simulink model "longModel_V0_1"  (R2023a)
settings: Solver=VariableStepAuto  StartTime=0.0  StopTime=100  RelTol=1e-3  AbsTol=1e-3
undefined symbols (not defined in the file or in its folder): STire
libraries: fl_lib x14, nesl_utility x10, sdl_lib x4, simulink x1
settings Model: Creator=Raheel Farouk  LastModifiedBy=Raheel Farouk
settings SolverCC: AutoScaleAbsTol=off  AlgebraicLoopSolver=TrustRegion  MaxZcPerStep=1
settings DebuggingCC: UnconnectedInputMsg=warning  UnconnectedOutputMsg=warning  UnconnectedLineMsg=warning  SymbolicDimsDataTypeCodeGenerationDiagnostic=none
settings ModelReferenceCC: EnableRefExpFcnMdlSchedulingChecks=on
settings SFSimCC: CustomCodeUndefinedFunction=UseInterfaceOnly
settings RTWCC: DLArmComputeVersion=19.05
settings SimscapeCC: SimscapeLogType=all  SimscapeLogSimulationStatistics=on  SimscapeLogDataHistory=10000

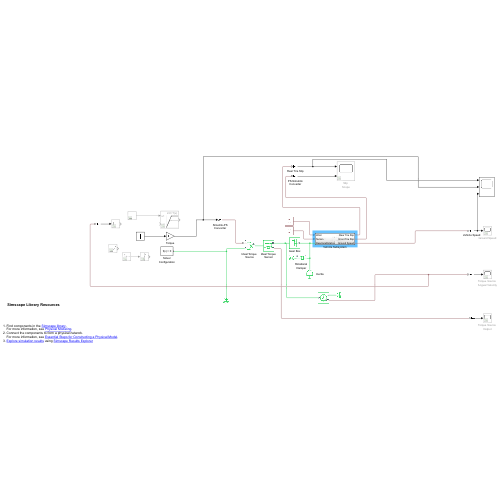
[thumbnail: Simulink's stored preview of the top-level diagram]
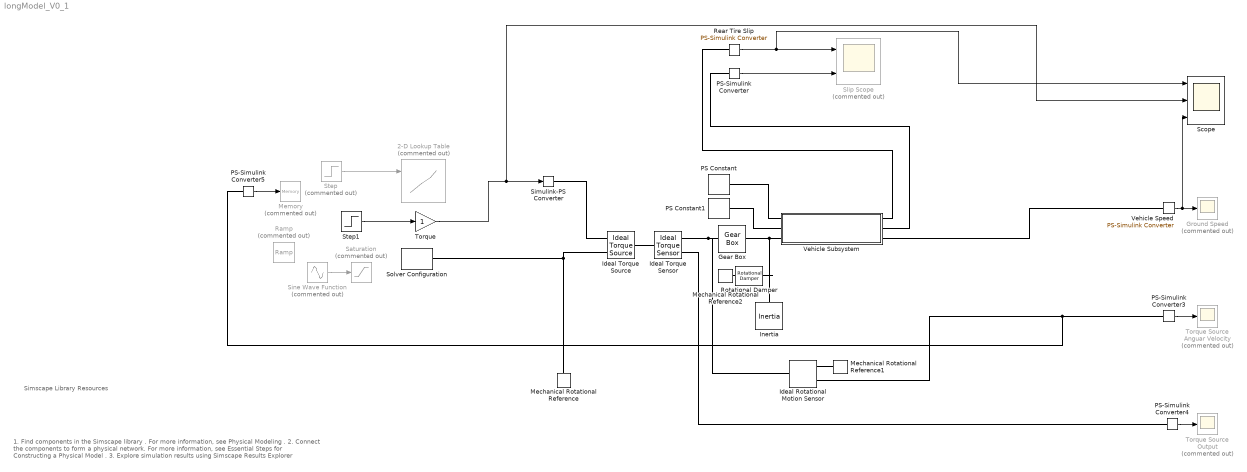
== system longModel_V0_1 ==
  note: 1. Find components in the Simscape library .
      | For more information, see Physical Modeling .
      | 2. Connect the components to form a physical network.
      | For more information, see Essential Steps for Constructing a Physical Model .
      | 3. Explore simulation results using Simscape Results Explorer
  note: Simscape Library Resources
  2-D Lookup Table : Lookup_n-D  Commented=on  BreakpointsForDimension1=[0;141;216.67;220;230;500]  BreakpointsForDimension2=[1;100;3321;5100]  Table=[0 0 0 0;141 141 141 141;216.67 216.67 216.67 141;220 220 216.67 141;220 230 216.67 141;220 230 216.67 141]  InternalRulePriority=Speed  RndMeth=Simplest
      settings: InputPortMap=u0,u1
  Gear Box : fl_lib/Mechanical/Mechanisms/Gear Box  ratio=3.15  t_in_specify=off  t_in_priority=None  t_in=0 N*m  t_in_nominal_specify=off  t_in_nominal_unit=N*m  t_in_nominal_value=1  t_out_specify=off  t_out_priority=None  t_out=0 N*m  t_out_nominal_specify=off  t_out_nominal_unit=N*m  t_out_nominal_value=1
  Ground Speed : Scope  Commented=on
  Ideal Rotational Motion Sensor : fl_lib/Mechanical/Mechanical Sensors/Ideal Rotational Motion Sensor  reference=foundation.enum.MeasurementReference.difference  acceleration_port=false  velocity_port=true  position_port=false  wrap_angle=false  offset=0 rad
      settings: InternalSimscapePortConfiguration="{\"Bottom\":[],\"Left\":[{\"id\":\"R\",\"label\":\"R\",\"type\":\"foundation.mechanical.rotational.rotational\"}],\"Right\":[{\"id\":\"C\",\"label\":\"C\",\"type\":\"foundation.mechanical.rotational.rotational\"},{\"id\":\"W\",\"label\":\"W\",\"type\":\"output\"}],\"Top\":[]}"
  Ideal Torque Sensor : fl_lib/Mechanical/Mechanical Sensors/Ideal Torque Sensor
  Ideal Torque Source : fl_lib/Mechanical/Mechanical Sources/Ideal Torque Source
  Inertia : fl_lib/Mechanical/Rotational Elements/Inertia  inertia=0.01 kg*m^2  num_ports=foundation.enum.numPorts2.one  w_specify=off  w_priority=High  w=0 rad/s  w_nominal_specify=off  w_nominal_unit=rad/s  w_nominal_value=1  t_specify=off  t_priority=None  t=0 N*m  t_nominal_specify=off  t_nominal_unit=N*m  t_nominal_value=1
  Mechanical Rotational Reference : fl_lib/Mechanical/Rotational Elements/Mechanical Rotational Reference
  Mechanical Rotational Reference1 : fl_lib/Mechanical/Rotational Elements/Mechanical Rotational Reference
  Mechanical Rotational Reference2 : fl_lib/Mechanical/Rotational Elements/Mechanical Rotational Reference
  Memory : Memory  Commented=on
  PS Constant : fl_lib/Physical Signals/Sources/PS Constant  constant=0
  PS Constant1 : fl_lib/Physical Signals/Sources/PS Constant  constant=0
  PS-Simulink Converter : nesl_utility/PS-Simulink Converter  PhysicalDomain=network_engine_domain  SubClassName=ps_output  LeftPortType=input  RightPortType=output  PseudoPeriodic=off  Frequencies=[]  VectorFormat=inherit  Unit=inherit  AffineConversion=off
  PS-Simulink Converter3 : nesl_utility/PS-Simulink Converter  PhysicalDomain=network_engine_domain  SubClassName=ps_output  LeftPortType=input  RightPortType=output  PseudoPeriodic=off  Frequencies=[]  VectorFormat=inherit  Unit=rpm  AffineConversion=off
  PS-Simulink Converter4 : nesl_utility/PS-Simulink Converter  PhysicalDomain=network_engine_domain  SubClassName=ps_output  LeftPortType=input  RightPortType=output  PseudoPeriodic=off  Frequencies=[]  VectorFormat=inherit  Unit=inherit  AffineConversion=off
  PS-Simulink Converter5 : nesl_utility/PS-Simulink Converter  PhysicalDomain=network_engine_domain  SubClassName=ps_output  LeftPortType=input  RightPortType=output  PseudoPeriodic=off  Frequencies=[]  VectorFormat=inherit  Unit=rpm  AffineConversion=off
  Ramp : simulink/Sources/Ramp  Commented=on  slope=10  start=5  InitialOutput=0
  Rear Tire Slip : nesl_utility/PS-Simulink Converter  PhysicalDomain=network_engine_domain  SubClassName=ps_output  LeftPortType=input  RightPortType=output  PseudoPeriodic=off  Frequencies=[]  VectorFormat=inherit  Unit=inherit  AffineConversion=off
  Rotational Damper : fl_lib/Mechanical/Rotational Elements/Rotational Damper  D=0.001 N*m*s/rad  w_specify=off  w_priority=None  w=0 rad/s  w_nominal_specify=off  w_nominal_unit=rad/s  w_nominal_value=1  t_specify=off  t_priority=None  t=0 N*m  t_nominal_specify=off  t_nominal_unit=N*m  t_nominal_value=1
  Saturation : Saturate  Commented=on  UpperLimit=300  LowerLimit=0
  Scope : Scope  NumInputPorts=3
  Simulink-PS Converter : nesl_utility/Simulink-PS Converter  PhysicalDomain=network_engine_domain  SubClassName=ps_input  LeftPortType=input  RightPortType=output  PseudoPeriodic=off  Frequencies=[]  NoiseDistribution=none  NoiseParameters=[]  Unit=1  AffineConversion=off  FilteringAndDerivatives=filter  SimscapeFilterOrder=1  InputFilterTimeConstant=0.001  UdotUserProvided=0
  Sine Wave Function : Sin  Commented=on  Bias=112  Frequency=0.4  SampleTime=0
  Slip Scope : Scope  Commented=on  NumInputPorts=2
  Solver Configuration : nesl_utility/Solver Configuration  PhysicalDomain=network_engine_domain  SubClassName=solver  LeftPortType=input  RightPortType=generic  Tones=[]  Harmonics=[]  SimulateNoise=off  Profile=off  UseLocalSampling=off  EnableSwitchedLinearOptims=on  FrequencyDomain=off  UseCCode=off  RelTol=0.001  AbsTol=1e-06  MinStep=1e-09  ToWorkspace=off  RevertToSquareIcSolve=off  NumHomotopyIterations=100  PhasorMode=off  PhasorModeNumHarmonics=1  ConsistencySolver=NEWTON_XTOL_AFTER_FTOL  IndexReductionMethod=DerivativeReplacement  DoDC=off  ResidualTolerance=1e-09  ConsistencyTolSource=GLOBAL  ConsistencyAbsTol=0.001  ConsistencyRelTol=0.001  ConsistencyTolFactor=0.001  UseLocalSolver=off  LocalSolverChoice=NE_BACKWARD_EULER_ADVANCER  ResolveIndetEquations=on  FunctionEvalNumThread=1  LocalSolverSampleTime=0.001  DoFixedCost=off  MaxNonlinIter=3  MaxModeIter=2  ComputeImpulses=off  ImpulseIterations=2  LinearAlgebra=auto  LinearAlgebraNumThread=0  EquationFormulation=NE_TIME_EF  DelaysMemoryBudget=1024  AutomaticFiltering=on  FilteringTimeConstant=0.001  PartitionStorageMethod=AS_NEEDED  PartitionMemoryBudget=1024  PartitionMethod=ROBUST
  Step : Step  Commented=on  Time=5  After=500  SampleTime=0
  Step1 : Step  Time=5  After=10  SampleTime=0
  Torque : Gain
  Torque Source Anguar Velocity : Scope  Commented=on
  Torque Source Output : Scope  Commented=on
  Vehicle Speed : nesl_utility/PS-Simulink Converter  PhysicalDomain=network_engine_domain  SubClassName=ps_output  LeftPortType=input  RightPortType=output  PseudoPeriodic=off  Frequencies=[]  VectorFormat=inherit  Unit=km/hr  AffineConversion=off
  Vehicle Subsystem : Subsystem
  wires:
  PS-Simulink Converter/1 -> Slip Scope/2
  Rear Tire Slip/1 -> Scope/1, Slip Scope/1
  Vehicle Speed/1 -> Scope/3, Ground Speed/1
  PS-Simulink Converter4/1 -> Torque Source Output/1
  PS-Simulink Converter3/1 -> Torque Source Anguar Velocity/1
  PS-Simulink Converter5/1 -> Memory/1
  Step/1 -> 2-D Lookup Table/1
  Sine Wave Function/1 -> Saturation/1
  Torque/1 -> Scope/2, Simulink-PS Converter/1
  Step1/1 -> Torque/1
  connections:
  Rear Tire Slip/LConn1 -- Vehicle Subsystem/RConn1
  Vehicle Subsystem/RConn2 -- PS-Simulink Converter/LConn1
  Vehicle Subsystem/RConn3 -- Vehicle Speed/LConn1
  Ideal Torque Source/RConn2 -- Solver Configuration/RConn1 -- Mechanical Rotational Reference/LConn1
  Ideal Torque Sensor/LConn1 -- Ideal Torque Source/LConn1
  PS-Simulink Converter4/LConn1 -- Ideal Torque Sensor/RConn2
  Ideal Rotational Motion Sensor/RConn1 -- Mechanical Rotational Reference1/LConn1
  Ideal Rotational Motion Sensor/RConn2 -- PS-Simulink Converter5/LConn1 -- PS-Simulink Converter3/LConn1
  PS Constant/RConn1 -- Vehicle Subsystem/LConn1
  PS Constant1/RConn1 -- Vehicle Subsystem/LConn2
  Ideal Rotational Motion Sensor/LConn1 -- Ideal Torque Sensor/RConn1 -- Gear Box/LConn1
  Vehicle Subsystem/LConn3 -- Rotational Damper/RConn1 -- Inertia/LConn1 -- Gear Box/RConn1
  Mechanical Rotational Reference2/LConn1 -- Rotational Damper/LConn1
  Simulink-PS Converter/RConn1 -- Ideal Torque Source/RConn1

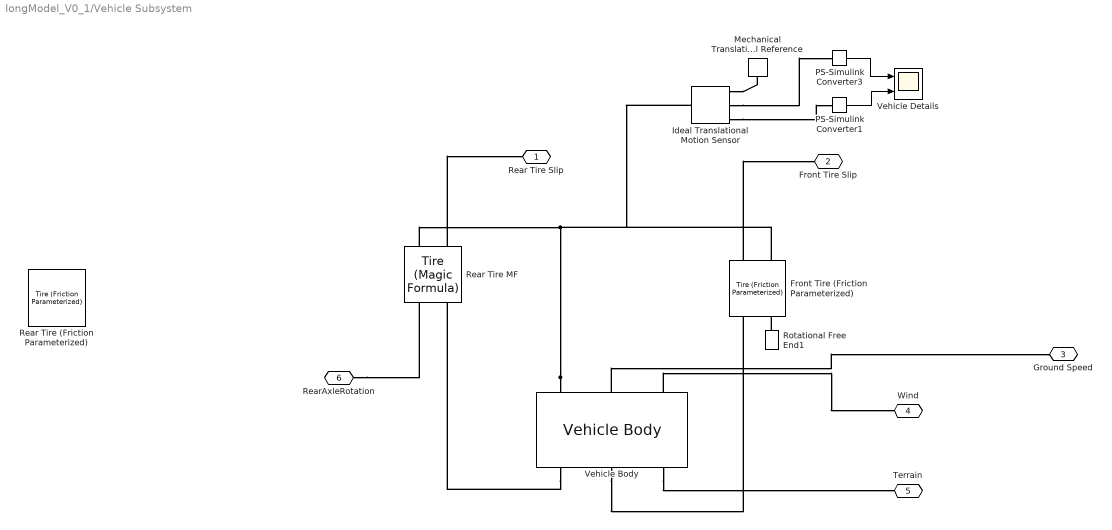
== system longModel_V0_1/Vehicle Subsystem ==
  Front Tire (Friction Parameterized) : sdl_lib/Tires & Vehicles/Tire (Friction Parameterized)  r_tire=508 mm  slip_output=sdl.enum.SlipOutput.Relative  friction_model=sdl.enum.friction_model_var.fixed  mu_static=0.9  mu_kinetic=0.7  slip_vector=[0, .02, .06, .15, .6, 1] rad/s  mu_kinetic_vector=[.89, .88, .8, .75, .7, .7]  interp_method=simscape.enum.interpolation.linear  extrap_method=simscape.enum.extrapolation.linear  model_compliance=sdl.enum.compliance.off  stiffness=1e6 N/m  damping=1000 N*s/m  model_inertia=sdl.enum.model_inertia.off  tire_inertia=1 kg*m^2  initial_velocity=0 rad/s  model_resistance=simscape.enum.onoff.off  resistance_model=sdl.enum.RollingResistance.Constant  coeff=0.015  p_tire=250e3 Pa  alpha=-0.003  beta=0.97  coeff_a=84e-4  coeff_b=6.2e-4 s/m  coeff_c=1.6e-4 s^2/m^2  v_thr=0.001 m/s  v_tol=0.01 m/s  F_min=10 N  initial_traction_state=sdl.enum.tireIC.traction
      settings: InternalSimscapePortConfiguration="{\"Bottom\":[],\"Left\":[{\"id\":\"N\",\"label\":\"N\",\"type\":\"input\"},{\"id\":\"A\",\"label\":\"A\",\"type\":\"foundation.mechanical.rotational.rotational\"}],\"Right\":[{\"id\":\"Srel\",\"label\":\"S\",\"type\":\"output\"},{\"id\":\"H\",\"label\":\"H\",\"type\":\"foundation.mechanical.translational.translational\"}],\"Top\":[]}"
  Ideal Translational Motion Sensor : fl_lib/Mechanical/Mechanical Sensors/Ideal Translational Motion Sensor  reference=foundation.enum.MeasurementReference.difference  acceleration_port=false  velocity_port=true  position_port=true  offset=0 m
  Mechanical Translational Reference : fl_lib/Mechanical/Translational Elements/Mechanical Translational Reference
  PS-Simulink Converter1 : nesl_utility/PS-Simulink Converter  PhysicalDomain=network_engine_domain  SubClassName=ps_output  LeftPortType=input  RightPortType=output  PseudoPeriodic=off  Frequencies=[]  VectorFormat=inherit  Unit=m  AffineConversion=off
  PS-Simulink Converter3 : nesl_utility/PS-Simulink Converter  PhysicalDomain=network_engine_domain  SubClassName=ps_output  LeftPortType=input  RightPortType=output  PseudoPeriodic=off  Frequencies=[]  VectorFormat=inherit  Unit=km/hr  AffineConversion=off
  Rear Tire (Friction Parameterized) : sdl_lib/Tires & Vehicles/Tire (Friction Parameterized)  r_tire=508 mm  slip_output=sdl.enum.SlipOutput.Relative  friction_model=sdl.enum.friction_model_var.fixed  mu_static=0.9  mu_kinetic=0.7  slip_vector=[0, .02, .06, .15, .6, 1] rad/s  mu_kinetic_vector=[.89, .88, .8, .75, .7, .7]  interp_method=simscape.enum.interpolation.linear  extrap_method=simscape.enum.extrapolation.linear  model_compliance=sdl.enum.compliance.off  stiffness=1e6 N/m  damping=1000 N*s/m  model_inertia=sdl.enum.model_inertia.off  tire_inertia=1 kg*m^2  initial_velocity=0 rad/s  model_resistance=simscape.enum.onoff.off  resistance_model=sdl.enum.RollingResistance.Constant  coeff=0.015  p_tire=250e3 Pa  alpha=-0.003  beta=0.97  coeff_a=84e-4  coeff_b=6.2e-4 s/m  coeff_c=1.6e-4 s^2/m^2  v_thr=0.001 m/s  v_tol=0.01 m/s  F_min=10 N  initial_traction_state=sdl.enum.tireIC.traction
      settings: InternalSimscapePortConfiguration="{\"Bottom\":[],\"Left\":[{\"id\":\"N\",\"label\":\"N\",\"type\":\"input\"},{\"id\":\"A\",\"label\":\"A\",\"type\":\"foundation.mechanical.rotational.rotational\"}],\"Right\":[{\"id\":\"Srel\",\"label\":\"S\",\"type\":\"output\"},{\"id\":\"H\",\"label\":\"H\",\"type\":\"foundation.mechanical.translational.translational\"}],\"Top\":[]}"
  Rear Tire MF : sdl_lib/Tires & Vehicles/Tire (Magic Formula)  parameterization=sdl.enum.magic_tire_model.peak  F_z1=3000 N  F_x1=3500 N  kappa1=10  B_m=10  C_m=1.9  D_m=1  E_m=0.97  fz0=STire.VERTICAL.FNOMIN N  p_Cx=STire.LONGITUDINAL_COEFFICIENTS.PCX  p_Dx=STire.LONGITUDINAL_COEFFICIENTS.PDX  p_Ex=STire.LONGITUDINAL_COEFFICIENTS.PEX  p_Kx=STire.LONGITUDINAL_COEFFICIENTS.PKX  p_Hx=STire.LONGITUDINAL_COEFFICIENTS.PHX  p_Vx=STire.LONGITUDINAL_COEFFICIENTS.PVX  rolling_radius_model=sdl.enum.RollingRadiusParameterization.MagicFormula  r_e=508 mm  r_0=STire.DIMENSION.UNLOADED_RADIUS m  breff=STire.VERTICAL.BREFF  dreff=STire.VERTICAL.DREFF  freff=STire.VERTICAL.FREFF  q_re0=STire.VERTICAL.Q_RE0  q_v1=STire.VERTICAL.Q_V1  longvl=STire.MODEL.LONGVL m/s  cz=STire.VERTICAL.VERTICAL_STIFFNESS N/m  model_resistance=true  resistance_model=sdl.enum.rollingResistanceParameterization.constant  coeff=0.015  p_tire=STire.OPERATING_CONDITIONS.INFLPRES Pa  alpha=-0.003  beta=0.97  coeff_a=84e-4  coeff_b=6.2e-4 s/m  coeff_c=1.6e-4 s^2/m^2  p_tire0=STire.OPERATING_CONDITIONS.NOMPRES Pa  fz0_resistance=STire.VERTICAL.FNOMIN N  vH0=STire.MODEL.LONGVL m/s  q_Sy=STire.ROLLING_COEFFICIENTS.QSY  v_thr=0.001 m/s  enable_scaling_coefficients=true  lfzO=STire.SCALING_COEFFICIENTS.LFZO  lcx=STire.SCALING_COEFFICIENTS.LCX  lmux=STire.SCALING_COEFFICIENTS.LMUX  lex=STire.SCALING_COEFFICIENTS.LEX  lkx=STire.SCALING_COEFFICIENTS.LKX  lhx=STire.SCALING_COEFFICIENTS.LHX  lvx=STire.SCALING_COEFFICIENTS.LVX  lmy=STire.SCALING_COEFFICIENTS.LMY  model_compliance=sdl.enum.compliance.off  stiffness=STire.STRUCTURAL.LONGITUDINAL_STIFFNESS N/m  damping=STire.STRUCTURAL.DAMP_LONG * sqrt(STire.INERTIA.MASS * STire.VERTICAL.FNOMIN / STire.DIMENSION.UNLOADED_RADIUS) N*s/m  model_inertia=sdl.enum.model_inertia.off  inertia=STire.INERTIA.IYY kg*m^2  initial_velocity=0 rad/s  vxlow=0.00001 m/s  v_tr_thr=0.1 m/s  kpumin=-2  kpumax=2
  Rotational Free End1 : fl_lib/Mechanical/Rotational Elements/Rotational Free End  w_specify=off  w_priority=None  w=0 rad/s  w_nominal_specify=off  w_nominal_unit=rad/s  w_nominal_value=1
  Vehicle Body : sdl_lib/Tires & Vehicles/Vehicle Body  mass=307 kg  n_w=2  x_f=864.45 mm  x_r=665.55 mm  y_c=330 mm  mass_var=simscape.enum.onoff.off  g=9.81 m/s^2  liftoff_warning=simscape.enum.onoff.off  area=3 m^2  Cd=0.4  rho=1.18 kg/m^3  model_pitch=simscape.enum.onoff.off  inertia=4000 kg*m^2  suspension_model=sdl.enum.linearTLU.linear  k_f=1e4 N/m  b_f=1e4 N*s/m  k_r=1e4 N/m  b_r=1e4 N*s/m  k_f_TLU=[-2000, -1000, 0, 1000, 2000] N  x_f_TLU=[-.4, -.2, 0, .2, .4] m  b_f_TLU=[-200, -100, 0, 100, 200] N  v_f_TLU=[-4, -2, 0, 2, 4] m/s  k_r_TLU=[-2000, -1000, 0, 1000, 2000] N  x_r_TLU=[-.4, -.2, 0, .2, .4] m  b_r_TLU=[-200, -100, 0, 100, 200] N  v_r_TLU=[-4, -2, 0, 2, 4] m/s  interp_method=simscape.enum.interpolation.linear  extrap_method=simscape.enum.extrapolation.linear  model_hardstop=simscape.enum.onoff.off  upper_bound_f=.25 m  lower_bound_f=-.25 m  stop_k_f=1e6 N/m  stop_b_f=150 N*s/m  upper_bound_r=.25 m  lower_bound_r=-.25 m  stop_k_r=1e6 N/m  stop_b_r=150 N*s/m  initial_pitch=0 rad  initial_pitch_rate=0 rad/s  v_specify=off  v_priority=High  v=0 m/s  v_nominal_specify=off  v_nominal_unit=m/s  v_nominal_value=1
  Vehicle Details : Scope  NumInputPorts=2
  Rear Tire Slip : PMIOPort  Side=Right
  Front Tire Slip : PMIOPort  Port=2  Side=Right
  Ground Speed : PMIOPort  Port=3  Side=Right
  Wind : PMIOPort  Port=4  Side=Left
  Terrain : PMIOPort  Port=5  Side=Left
  RearAxleRotation : PMIOPort  Port=6  Side=Left
  wires:
  PS-Simulink Converter3/1 -> Vehicle Details/1
  PS-Simulink Converter1/1 -> Vehicle Details/2
  connections:
  RearAxleRotation/RConn1 -- Rear Tire MF/LConn2
  Vehicle Body/LConn1 -- Rear Tire MF/RConn2 -- Ideal Translational Motion Sensor/LConn1 -- Front Tire (Friction Parameterized)/RConn2
  Vehicle Body/LConn3 -- Wind/RConn1
  Vehicle Body/RConn3 -- Terrain/RConn1
  Vehicle Body/RConn1 -- Rear Tire MF/LConn1
  Rotational Free End1/LConn1 -- Front Tire (Friction Parameterized)/LConn2
  Vehicle Body/RConn2 -- Front Tire (Friction Parameterized)/LConn1
  Front Tire (Friction Parameterized)/RConn1 -- Front Tire Slip/RConn1
  Rear Tire MF/RConn1 -- Rear Tire Slip/RConn1
  Vehicle Body/LConn2 -- Ground Speed/RConn1
  Ideal Translational Motion Sensor/RConn1 -- Mechanical Translational Reference/LConn1
  Ideal Translational Motion Sensor/RConn2 -- PS-Simulink Converter3/LConn1
  Ideal Translational Motion Sensor/RConn3 -- PS-Simulink Converter1/LConn1
